simulink model "HB_FB_1ph_inverter"  (R2022b)
settings: Solver=FixedStepDiscrete  StartTime=0.0  StopTime=0.1  MaxStep=Ts  RelTol=1e-3
InitFcn:
  | clear;
  | clc;
  | Ts=1/50/3240;
  | clc;
libraries: spsIGBTDiodeLib x6, spsGroundLib x4, spsDCVoltageSourceLib x3, spsSeriesRLCBranchLib x2, spsCurrentMeasurementLib x2, simulink x2, spsVoltageMeasurementLib x2, sps_lib x1
Description:
  | Copyright 2008 The MathWorks(TM), Inc.
settings Model: Creator=patrice  LastModifiedBy=Hadi
settings SolverCC: AlgebraicLoopSolver=TrustRegion
settings DataIOCC: SaveFormat=Array  SignalLoggingSaveFormat=ModelDataLogs  ReturnWorkspaceOutputs=off  SignalLoggingName=sigsOut
settings OptimizationCC: BlockReduction=off  BooleanDataType=off  ExpressionDepthLimit=2147483647  InitFltsAndDblsToZero=on  EfficientMapNaN2IntZero=off  LifeSpan=inf
settings DebuggingCC: SaveWithParameterizedLinksMsg=none  UnderspecifiedInitializationDetection=Classic  MergeDetectMultiDrivingBlocksExec=none  CheckExecutionContextPreStartOutputMsg=on  SignalResolutionControl=TryResolveAllWithWarning  MultiTaskDSMMsg=warning  MultiTaskCondExecSysMsg=none  FcnCallInpInsideContextMsg=warning  UnconnectedInputMsg=warning  UnconnectedOutputMsg=warning  UnconnectedLineMsg=warning  StateNameClashWarn=warning  SFUnexpectedBacktrackingDiag=warning  SFNoUnconditionalDefaultTransitionDiag=warning  SFExecutionAtInitializationDiag=none  SFMachineParentedDataDiag=warning  ArithmeticOperatorsInVariantConditions=warning
settings HardwareCC: ProdBitPerPointer=32  ProdBitPerSizeT=32  ProdBitPerPtrDiffT=32  ProdLargestAtomicFloat=None  ProdIntDivRoundTo=Undefined  ProdEndianess=Unspecified  ProdWordSize=32  ProdHWDeviceType=32-bit Generic  TargetUnknown=on
settings ModelReferenceCC: PropagateSignalLabelsOutOfModel=off
settings SFSimCC: SimUseLocalCustomCode=off  CustomCodeUndefinedFunction=UseInterfaceOnly
settings RTWCC: RTWUseLocalCustomCode=off
settings CodeAppCC: StateflowObjectComments=on
settings GRTTargetCC: TargetFcnLib=ansi_tfl_tmw.mat  TargetLangStandard=C89/C90 (ANSI)  CombineOutputUpdateFcns=off  GRTInterface=on
settings ConfigComp: CovMetricSettings=dw  CovSaveCumulativeToWorkspaceVar=on  CovSaveSingleToWorkspaceVar=on  CovExternalEMLEnable=off

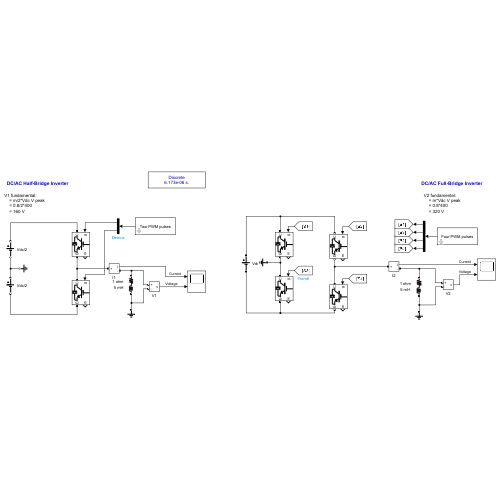
[thumbnail: Simulink's stored preview of the top-level diagram]
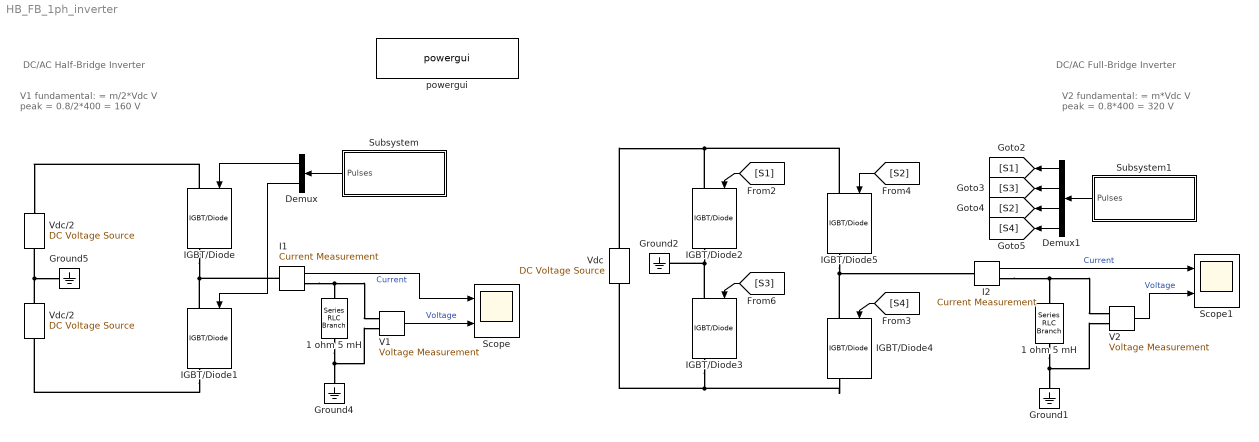
== system HB_FB_1ph_inverter ==
  note: V1 fundamental:
      |     = m/2*Vdc V peak
      |     = 0.8/2*400
      |     = 160 V
  note: DC/AC Half-Bridge Inverter
  note: DC/AC Full-Bridge Inverter
  note: V2 fundamental:
      |     = m*Vdc V peak
      |     = 0.8*400
      |     = 320 V
  1 ohm 5 mH : spsSeriesRLCBranchLib/Series RLC Branch  LConnTagsString=__new0  RConnTagsString=__new0  BranchType=RL  Resistance=1  Inductance=5e-03  SetiL0=off  InitialCurrent=0  Capacitance=[]  Setx0=off  InitialVoltage=0  Measurements=None
  "1 ohm 5 mH " : spsSeriesRLCBranchLib/Series RLC Branch  LConnTagsString=__new0  RConnTagsString=__new0  BranchType=RL  Resistance=1  Inductance=5e-03  SetiL0=off  InitialCurrent=0  Capacitance=[]  Setx0=off  InitialVoltage=0  Measurements=None
  Demux : Demux  Outputs=2
  Demux1 : Demux
  Ground{1..2,4..5} (4 alike) : spsGroundLib/Ground  LConnTagsString=a
  I1 : spsCurrentMeasurementLib/Current Measurement  Tag=PoWeRsYsTeMmEaSuReMeNt  PhasorSimulation=off  OutputType=Magnitude  PSBequivalent=0
      settings: AttributesFormatString=\n
  I2 : spsCurrentMeasurementLib/Current Measurement  Tag=PoWeRsYsTeMmEaSuReMeNt  PhasorSimulation=off  OutputType=Magnitude  PSBequivalent=0
      settings: AttributesFormatString=\n
  IGBT/Diode{,1..5} (6 alike) : spsIGBTDiodeLib/IGBT//Diode  Ron=1e-3  Rs=1e5  Cs=inf  Measurements=on
  Scope : Scope  NumInputPorts=2
  Scope1 : Scope  NumInputPorts=2
  Subsystem : Subsystem  mask(PWM Generator){modulation_index=0.8, Fc=1080, f=50, Phase=0, Ts=Ts}
      mask prompts: modulation_index "Modulation Index"; Fc "Switching Frequency"; f "Output Frequency"; Ts "Sampling Time"
      mask help:
      | This module generates two sinosoidal PWM pulses for half bridge inverter.
      |
      | Syed Abdul Rahman Kashif
      | UET Lahore
      mask Display: fprintf('Two PWM pulses')
  Subsystem1 : Subsystem  mask(PWM Generator){modulation_index=0.8, Fc=1080, f=50, Phase=0, Ts=Ts}
      mask prompts: modulation_index "Modulation Index"; Fc "Switching Frequency"; f "Output Frequency"; Ts "Sampling Time"
      mask help:
      | This module generates four sinosoidal PWM pulses for full bridge inverter.
      |
      | Syed Abdul Rahman Kashif
      | UET Lahore
      mask Display: fprintf('Four PWM pulses')
  V1 : spsVoltageMeasurementLib/Voltage Measurement  Tag=PoWeRsYsTeMmEaSuReMeNt  PhasorSimulation=off  OutputType=Magnitude  PSBequivalent=0
  V2 : spsVoltageMeasurementLib/Voltage Measurement  Tag=PoWeRsYsTeMmEaSuReMeNt  PhasorSimulation=off  OutputType=Magnitude  PSBequivalent=0
  Vdc : spsDCVoltageSourceLib/DC Voltage Source  Description=source block  Amplitude=400  Measurements=None
      settings: AttributesFormatString=\n
  Vdc/2 : spsDCVoltageSourceLib/DC Voltage Source  Description=source block  Amplitude=200  Measurements=None
      settings: AttributesFormatString=\n
  "Vdc/2 " : spsDCVoltageSourceLib/DC Voltage Source  Description=source block  Amplitude=200  Measurements=None
      settings: AttributesFormatString=\n
  powergui : sps_lib/powergui  SimulationMode=Discrete  SampleTime=Ts  frequency=60  Iterations=50  frequencyindice=0  Pbase=100e6  ErrMax=1e-4  UnitsV=kV  UnitsW=MW  buscounter=0  FunctionMessages=off  echomessages=off  EnableUseOfTLC=off  CurrentSourceSwitches=off  DisableSnubberDevices=off  DisableRonSwitches=off  DisableVfSwitches=off  DisplayEquations=off  AutomaticDiscreteSolvers=off  SolverType=Tustin/Backward Euler (TBE)  Interpol=off  ExternalGateDelay=off  methode=off  Ts=0  x0status=blocks  SPID=off  SwTol=0  HookPort=off  NonlinearTolerance=1e-4  nMaxIteration=100  ContinueOnMaxIteration=off  RestoreLinks=warning  ResistiveCurrentMeasurement=off  Frange=[0:2:500]  Ylog=off  Xlog=on  ShowGrid=off  save=off  variable=ZData  structure=Half_bridge_VI  ZoomFFT=off  StartTime=0.04  cycles=2  DisplayStyle=2  fundamental=50  FreqAxis=off  MaxFrequency=5000  frequencyindicesteady=1  RmsSteady=1  display=off
  wires:
  I1/1 -> Scope/1  "Current"
  V1/1 -> Scope/2  "Voltage"
  Subsystem/1(Pulses) -> Demux/1
  Demux/1 -> IGBT/Diode/1
  Demux/2 -> IGBT/Diode1/1
  I2/1 -> Scope1/1  "Current"
  V2/1 -> Scope1/2  "Voltage"
  Subsystem1/1(Pulses) -> Demux1/1
  Demux1/1 -> [S1]
  Demux1/2 -> [S3]
  [S1] -> IGBT/Diode2/1
  [S3] -> IGBT/Diode3/1
  Demux1/3 -> [S2]
  Demux1/4 -> [S4]
  [S2] -> IGBT/Diode5/1
  [S4] -> IGBT/Diode4/1
  connections:
  "Vdc/2 "/RConn1 -- Ground5/LConn1 -- Vdc/2/LConn1
  1 ohm 5 mH/RConn1 -- Ground4/LConn1 -- V1/LConn2
  IGBT/Diode1/RConn1 -- "Vdc/2 "/LConn1
  IGBT/Diode/LConn1 -- Vdc/2/RConn1
  I2/RConn1 -- "1 ohm 5 mH "/LConn1 -- V2/LConn1
  "1 ohm 5 mH "/RConn1 -- Ground1/LConn1 -- V2/LConn2
  IGBT/Diode3/RConn1 -- IGBT/Diode4/RConn1 -- Vdc/LConn1
  Vdc/RConn1 -- IGBT/Diode2/LConn1 -- IGBT/Diode5/LConn1
  I1/LConn1 -- IGBT/Diode1/LConn1 -- IGBT/Diode/RConn1
  IGBT/Diode2/RConn1 -- Ground2/LConn1 -- IGBT/Diode3/LConn1
  IGBT/Diode4/LConn1 -- IGBT/Diode5/RConn1 -- I2/LConn1
  1 ohm 5 mH/LConn1 -- I1/RConn1 -- V1/LConn1

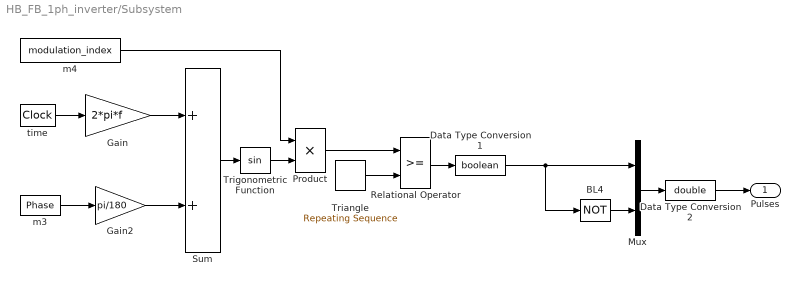
== system HB_FB_1ph_inverter/Subsystem ==
  BL4 : Logic  Operator=NOT  Inputs=1  SampleTime=Ts
  Data Type Conversion1 : DataTypeConversion  OutDataTypeStr=boolean  SampleTime=Ts
  Data Type Conversion2 : DataTypeConversion  OutDataTypeStr=double  SampleTime=Ts
  Gain : Gain  Gain=2*pi*f  SaturateOnIntegerOverflow=on  OutDataTypeStr=Inherit: Same as input  ParamDataTypeStr=Inherit: Same as input
  Gain2 : Gain  Gain=pi/180  SaturateOnIntegerOverflow=on  OutDataTypeStr=Inherit: Same as input  ParamDataTypeStr=Inherit: Same as input
  Mux : Mux  Inputs=2
  Product : Product  InputSameDT=on  SaturateOnIntegerOverflow=on  SampleTime=Ts  OutDataTypeStr=Inherit: Same as first input
  Relational Operator : RelationalOperator  SampleTime=Ts
  Sum : Sum  InputSameDT=on  SaturateOnIntegerOverflow=on  SampleTime=Ts  OutDataTypeStr=Inherit: Same as first input
  Triangle : simulink/Sources/Repeating Sequence  rep_seq_t=[0 1/Fc/4 3/Fc/4 1/Fc]  rep_seq_y=[0 -1 1 0]
  Trigonometric Function : Trigonometry  SampleTime=Ts
  m3 : Constant  Value=Phase  SampleTime=Ts
  m4 : Constant  Value=modulation_index  SampleTime=Ts
  time : DigitalClock  SampleTime=Ts
  Pulses : Outport  SampleTime=Ts
  wires:
  BL4/1 -> Mux/2
  Triangle/1 -> Relational Operator/2
  Product/1 -> Relational Operator/1
  Trigonometric Function/1 -> Product/2
  Sum/1 -> Trigonometric Function/1
  m4/1 -> Product/1
  m3/1 -> Gain2/1
  Gain2/1 -> Sum/2
  Gain/1 -> Sum/1
  time/1 -> Gain/1
  Relational Operator/1 -> Data Type Conversion1/1
  Data Type Conversion1/1 -> BL4/1, Mux/1
  Mux/1 -> Data Type Conversion2/1
  Data Type Conversion2/1 -> Pulses/1

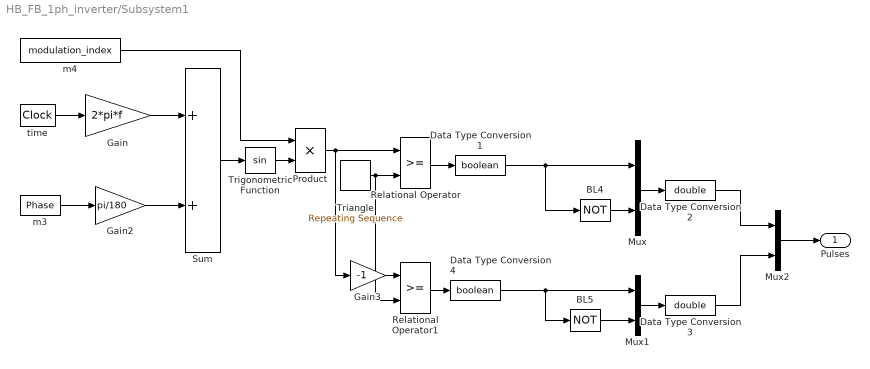
== system HB_FB_1ph_inverter/Subsystem1 ==
  BL4 : Logic  Operator=NOT  Inputs=1  SampleTime=Ts
  BL5 : Logic  Operator=NOT  Inputs=1  SampleTime=Ts
  Data Type Conversion1 : DataTypeConversion  OutDataTypeStr=boolean  SampleTime=Ts
  Data Type Conversion2 : DataTypeConversion  OutDataTypeStr=double  SampleTime=Ts
  Data Type Conversion3 : DataTypeConversion  OutDataTypeStr=double  SampleTime=Ts
  Data Type Conversion4 : DataTypeConversion  OutDataTypeStr=boolean  SampleTime=Ts
  Gain : Gain  Gain=2*pi*f  SaturateOnIntegerOverflow=on  OutDataTypeStr=Inherit: Same as input  ParamDataTypeStr=Inherit: Same as input
  Gain2 : Gain  Gain=pi/180  SaturateOnIntegerOverflow=on  OutDataTypeStr=Inherit: Same as input  ParamDataTypeStr=Inherit: Same as input
  Gain3 : Gain  Gain=-1  SaturateOnIntegerOverflow=on  SampleTime=Ts  OutDataTypeStr=Inherit: Same as input  ParamDataTypeStr=Inherit: Same as input
  Mux : Mux  Inputs=2
  Mux1 : Mux  Inputs=2
  Mux2 : Mux  Inputs=2
  Product : Product  InputSameDT=on  SaturateOnIntegerOverflow=on  SampleTime=Ts  OutDataTypeStr=Inherit: Same as first input
  Relational Operator : RelationalOperator  SampleTime=Ts
  Relational Operator1 : RelationalOperator  SampleTime=Ts
  Sum : Sum  InputSameDT=on  SaturateOnIntegerOverflow=on  SampleTime=Ts  OutDataTypeStr=Inherit: Same as first input
  Triangle : simulink/Sources/Repeating Sequence  rep_seq_t=[0 1/Fc/4 3/Fc/4 1/Fc]  rep_seq_y=[0 -1 1 0]
  Trigonometric Function : Trigonometry  SampleTime=Ts
  m3 : Constant  Value=Phase  SampleTime=Ts
  m4 : Constant  Value=modulation_index  SampleTime=Ts
  time : DigitalClock  SampleTime=Ts
  Pulses : Outport  SampleTime=Ts
  wires:
  Data Type Conversion2/1 -> Mux2/1
  Mux/1 -> Data Type Conversion2/1
  Data Type Conversion1/1 -> Mux/1, BL4/1
  Relational Operator/1 -> Data Type Conversion1/1
  time/1 -> Gain/1
  Gain/1 -> Sum/1
  Gain2/1 -> Sum/2
  m3/1 -> Gain2/1
  m4/1 -> Product/1
  Sum/1 -> Trigonometric Function/1
  Trigonometric Function/1 -> Product/2
  Product/1 -> Relational Operator/1, Gain3/1
  Triangle/1 -> Relational Operator/2, Relational Operator1/2
  BL4/1 -> Mux/2
  Mux1/1 -> Data Type Conversion3/1
  BL5/1 -> Mux1/2
  Gain3/1 -> Relational Operator1/1
  Relational Operator1/1 -> Data Type Conversion4/1
  Data Type Conversion4/1 -> BL5/1, Mux1/1
  Data Type Conversion3/1 -> Mux2/2
  Mux2/1 -> Pulses/1
